simulink model "simulink_model"  (R2024a)
settings: Solver=VariableStepAuto  StartTime=0.0  StopTime=0.5  RelTol=1e-3
libraries: cstblocks x2
settings Model: Creator=Yoru  LastModifiedBy=Yoru

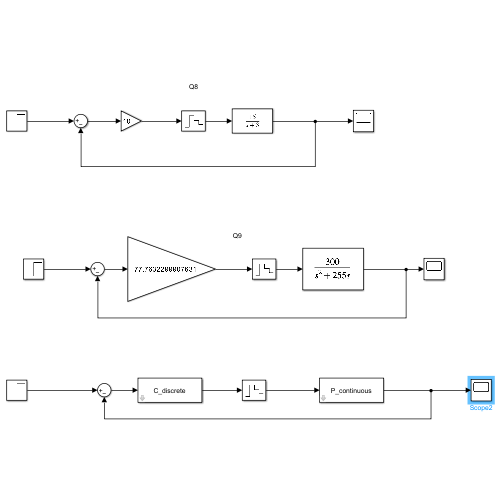
[thumbnail: Simulink's stored preview of the top-level diagram]
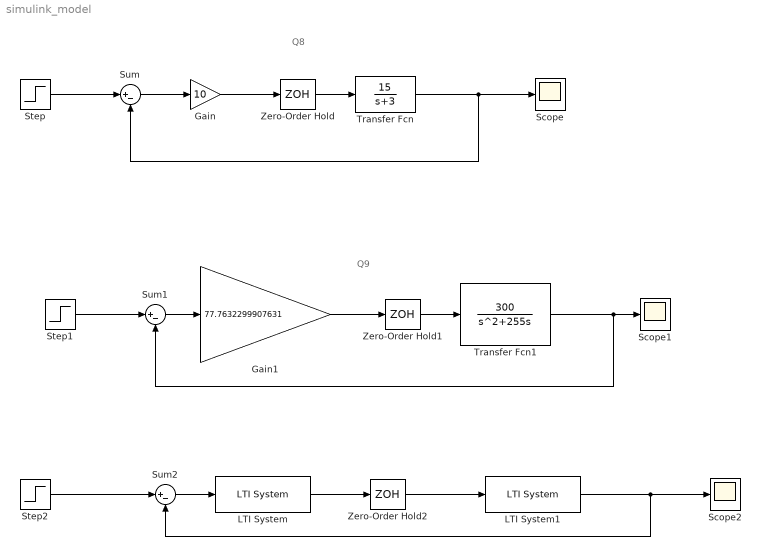
== system simulink_model ==
  note: Q8
  note: Q9
  Gain : Gain  Gain=10
  Gain1 : Gain  Gain=77.7632299907631
  LTI System : cstblocks/LTI System  sys=C_discrete  IC=[]  PadeOrder=0
  LTI System1 : cstblocks/LTI System  sys=P_continuous  IC=[]  PadeOrder=0
  Scope : Scope
  Scope1 : Scope
  Scope2 : Scope
  Step : Step  Time=0  SampleTime=0
  Step1 : Step  Time=0  SampleTime=0
  Step2 : Step  Time=0.1  After=1000  SampleTime=0
  Sum : Sum  Inputs=|+-
  Sum1 : Sum  Inputs=|+-
  Sum2 : Sum  Inputs=|+-
  Transfer Fcn : TransferFcn  Numerator=[15]  Denominator=[1 3]
  Transfer Fcn1 : TransferFcn  Numerator=[300]  Denominator=[1 255 0]
  Zero-Order Hold : ZeroOrderHold  SampleTime=0.008
  Zero-Order Hold1 : ZeroOrderHold  SampleTime=0.005
  Zero-Order Hold2 : ZeroOrderHold  SampleTime=1e-3
  wires:
  Step/1 -> Sum/1
  Sum/1 -> Gain/1
  Gain/1 -> Zero-Order Hold/1
  Zero-Order Hold/1 -> Transfer Fcn/1
  Transfer Fcn/1 -> Sum/2, Scope/1
  Transfer Fcn1/1 -> Sum1/2, Scope1/1
  Step1/1 -> Sum1/1
  Zero-Order Hold1/1 -> Transfer Fcn1/1
  Gain1/1 -> Zero-Order Hold1/1
  Sum1/1 -> Gain1/1
  Step2/1 -> Sum2/1
  Sum2/1 -> LTI System/1
  LTI System/1 -> Zero-Order Hold2/1
  Zero-Order Hold2/1 -> LTI System1/1
  LTI System1/1 -> Sum2/2, Scope2/1
